simulink library "tqd"  (R2021b)
settings: Solver=VariableStepAuto  StartTime=0.0  StopTime=10.0  RelTol=1e-3
undefined symbols (not defined in the file): ATQD_AfterTqMinGain_X_Deg, ATQD_APSCreepBaseTqD_X_kph, ATQD_APSCreepBaseTqD_Y_Deg, ATQD_APSCreepBaseTqR_X_kph, ATQD_APSCreepBaseTqR_Y_Deg, ATQD_APSCreepIterm_X_kph, ATQD_APSCreepIterm_Y_kph, ATQD_APSCreepPterm_X_kph, ATQD_APSCreepPterm_Y_kph, ATQD_APSDecReq_X_kph, ATQD_APSDecReq_Y_mps2, ATQD_APSDecReqCMD_X_kph, ATQD_APSDecReqTs_X_pct, ATQD_APSDecTimeGain_X_Deg, ATQD_APSDecTimeGain_Y_s, ATQD_APSReqLowSpd_X_Deg, ATQD_AutoHoldReleaseBPS_X_Deg, ATQD_AWDLoadTrqnsGain_X_kg, ATQD_AWDLoadTrqnsGain_Y_pct, ATQD_BOSEnBPSPosn_X_kph, ATQD_BOSMap_X_rpm, ATQD_BOSMap_Y_pct, ATQD_CreepBaseTqD_X_kph, ATQD_CreepBaseTqD_Y_Deg, ATQD_CreepBaseTqR_X_kph, ATQD_CreepBaseTqR_Y_Deg, ATQD_CreepBPSDisPosn_X_Deg, ATQD_CreepBPSDisPosnR_X_Deg, ATQD_CreepBPSEnPosn_X_Deg, ATQD_CreepBPSEnPosnR_X_Deg, ATQD_CreepDeltaTq_X_kph, ATQD_CreepIterm_X_kph, ATQD_CreepIterm_Y_kph, ATQD_CreepItermMaxLimit_X_pct, ATQD_CreepPreloadTime_X_kph, ATQD_CreepPreloadTq_X_kph, ATQD_CreepPreloadTq_Y_s, ATQD_CreepProtTq_X_Deg, ATQD_CreepPterm_X_kph, ATQD_CreepPterm_Y_kph, ATQD_CreepRrTqSpRat_X_rpm, ATQD_CreepRrTqSpRat_Y_Nm, ATQD_CreepTargetSpdD_X_pct, ATQD_CreepTargetSpdR_X_pct, ATQD_ECOTqMapD_X_rpm, ATQD_ECOTqMapD_Y_pct, ATQD_EMTqMapD_X_rpm, ATQD_EMTqMapD_Y_pct, ATQD_EOPDTqMapDCon_X_rpm, ATQD_EOPDTqMapDCon_Y_Deg, ATQD_EscapeModePedTq_X_pct, ATQD_EscapeModePedTq_Y_rpm, ATQD_EscapeModePedTqFr_X_pct, ATQD_EscapeModePedTqFr_Y_rpm, ATQD_EstInitVehWeight_X_c, ATQD_FAfterTqCMDGain_X_rpm, ATQD_FAfterTqCMDGain_Y_pct, ATQD_FrLossMAPLowV_X_rpm, ATQD_FrLossMAPLowV_Y_Nm, ATQD_FrMotActReduce_X_rpm ... (+772)
libraries: simulink x211, hcu_lib x179, tqr x3
(part 27 of 28)

== stateflow chart tqd/TQD/TorqueDemand/Signal_convert/SWC_Subsystem/Speed Control Mode ==
  state OFF
    en:
    VTQD_SpdCtrlMode_enum = ENUM_SPDCTRLMODE_OFF;
    VTQD_SpdCtrlSta_flg = FALSE;
  state ACC
    en:
    VTQD_SpdCtrlMode_enum = ENUM_SPDCTRLMODE_ACC;
    VTQD_SpdCtrlSta_flg = TRUE;
  state CC
    en:
    VTQD_SpdCtrlMode_enum = ENUM_SPDCTRLMODE_CC;
    VTQD_SpdCtrlSta_flg = TRUE;
  state MSA
    en:
    VTQD_SpdCtrlMode_enum = ENUM_SPDCTRLMODE_MSA;
    VTQD_SpdCtrlSta_flg = TRUE;
  state ISA
    en:
    VTQD_SpdCtrlMode_enum = ENUM_SPDCTRLMODE_ISA;
    VTQD_SpdCtrlSta_flg = TRUE;
  (default) -> OFF
  OFF -> (junction 29) [order 2]
  (junction 29) -> (junction 31) : [
      | VPMM_PowerSta_enum == ENUM_POWERSTA_READY &&...
      | VTQD_ShiftGearPosn_enum == ENUM_GEARPOSNTOCAN_D &&...
      | VINP_ADASACCSta_enum != ENUM_ADASACCSTA_OFF &&...
      | VTQD_SpdCtrlShortP_flg]
  (junction 26) -> (junction 93)
  (junction 100) -> (junction 26)
  (junction 40) -> OFF
  (junction 93) -> (junction 40)
  (junction 38) -> (junction 40)
  (junction 36) -> (junction 93)
  OFF -> ACC [order 1] : [
      | VPMM_PowerSta_enum == ENUM_POWERSTA_READY &&...
      | VTQD_ShiftGearPosn_enum == ENUM_GEARPOSNTOCAN_D &&...
      | VINP_ADASACCSta_enum == ENUM_ADASACCSTA_OFF && ...
      | VTQD_SpdCtrlShortP_flg
      | ]
  ACC -> (junction 38) [order 1] : [
      | VPMM_PowerSta_enum != ENUM_POWERSTA_READY ||...
      | VTQD_ShiftGearPosn_enum != ENUM_GEARPOSNTOCAN_D ||...
      | (VINP_ADASACCSta_enum == ENUM_ADASACCSTA_DISABLE ||...
      | VINP_ADASACCSta_enum == ENUM_ADASACCSTA_ERROR) ||...
      | VTQD_SpdCtrlLongP_flg
      | ]
  ACC -> CC [order 2] : [VTQD_SpdCtrlShortP_flg]
  CC -> (junction 36) [order 1] : [
      | VPMM_PowerSta_enum != ENUM_POWERSTA_READY||...
      | VTQD_ShiftGearPosn_enum != ENUM_GEARPOSNTOCAN_D ||...
      | VTQD_SpdCtrlLongP_flg
      | ]
  (junction 31) -> CC
  CC -> (junction 11) [order 2]
  (junction 11) -> (junction 14) [order 2]
  (junction 11) -> MSA [order 1] : [
      | VTQD_SpdCtrlShortP_flg && ...
      | (VINP_ADASISASta_enum == ENUM_ADASISASTA_DISABLE ||...
      | VINP_ADASISASta_enum == ENUM_ADASISASTA_ERROR || ...
      | !VTQD_IVIISAOffsetSpdCHOOSE_flg)
      | %add20230704
      | ]
  (junction 14) -> ISA : [
      | VTQD_SpdCtrlShortP_flg && ...
      | VINP_ADASISASta_enum == ENUM_ADASISASTA_OFF  && ...
      | VTQD_IVIISAOffsetSpdCHOOSE_flg
      | %add20230704
      | ]
  MSA -> ISA [order 2] : [
      | VINP_ADASISASta_enum == ENUM_ADASISASTA_OFF  && ...
      | VTQD_IVIISAOffsetSpdCHOOSE_flg
      | ]
  ISA -> (junction 100) [order 2] : [
      | VINP_ADASISASta_enum == ENUM_ADASISASTA_ERROR || ...
      | VINP_ADASISASta_enum == ENUM_ADASISASTA_DISABLE || ...
      | !VTQD_IVIISAOffsetSpdCHOOSE_flg
      | ]
  (junction 24) -> (junction 100)
  MSA -> (junction 19) [order 1]
  ISA -> (junction 21) [order 1]
  (junction 19) -> (junction 21)
  (junction 21) -> (junction 24) : [VPMM_PowerSta_enum != ENUM_POWERSTA_READY || ...
      | VTQD_ShiftGearPosn_enum != ENUM_GEARPOSNTOCAN_D ||...
      | VTQD_SpdCtrlShortP_flg || ...
      | VTQD_SpdCtrlLongP_flg
      | ]
  data: VPMM_PowerSta_enum input; VTQD_SpdCtrlShortP_flg input; VTQD_SpdCtrlLongP_flg input; ENUM_SPDCTRLMODE_OFF parameter; ENUM_SPDCTRLMODE_ACC parameter; ENUM_SPDCTRLMODE_CC parameter; ENUM_SPDCTRLMODE_ISA parameter; ENUM_SPDCTRLMODE_MSA parameter; FALSE parameter; ENUM_ADASACCSTA_DISABLE parameter; VINP_ADASACCSta_enum input; ENUM_POWERSTA_READY parameter; VINP_ADASISASta_enum input; ENUM_ADASISASTA_DISABLE parameter; VTQD_SpdCtrlMode_enum output uint8; VTQD_SpdCtrlSta_flg output boolean; TRUE parameter; VTQD_IVIISAOffsetSpdCHOOSE_flg input; ENUM_ADASISASTA_ERROR parameter; ENUM_ADASISASTA_OFF parameter; ENUM_ADASACCSTA_ERROR parameter; ENUM_ADASACCSTA_OFF parameter; VTQD_ShiftGearPosn_enum input; ENUM_GEARPOSNTOCAN_D parameter

== stateflow chart tqd/TQD/TorqueDemand/Signal_convert/Regen Level Switch ==
  state OFF
    en:
    VTQD_RegenMode_enum = ENUM_REGENLEVEL_OFF;
  state UserSetting
  state Lv1
    en:
    VTQD_RegenMode_enum = ENUM_REGENLEVEL_LV1;
    VTQD_SaveRegenMode_enum = ENUM_REGENLEVEL_LV1;
  state Lv2
    en:
    VTQD_RegenMode_enum = ENUM_REGENLEVEL_LV2;
    VTQD_SaveRegenMode_enum = ENUM_REGENLEVEL_LV2;
  state Lv3
    en:
    VTQD_RegenMode_enum = ENUM_REGENLEVEL_LV3;
    VTQD_SaveRegenMode_enum = ENUM_REGENLEVEL_LV3;
  state Lv4
    en:
    VTQD_RegenMode_enum = ENUM_REGENLEVEL_LV4;
    VTQD_SaveRegenMode_enum = ENUM_REGENLEVEL_LV4;
  state Lv5
    en:
    VTQD_RegenMode_enum = ENUM_REGENLEVEL_LV5;
    VTQD_SaveRegenMode_enum = ENUM_REGENLEVEL_LV5;
  state One_Pedal_Drive_Mode
    en:
    VTQD_RegenMode_enum = ENUM_REGENLEVEL_OPD;
    VTQD_SaveRegenMode_enum = ENUM_REGENLEVEL_OPD;
  (default) -> OFF : {
      | VTQD_SaveRegenMode_enum = VTQD_ReadRegenMode_enum;
      | }
  Lv1 -> (junction 102) [order 3] : [(VTQD_RegenSWSta_enum == ...
      | ENUM_REGENSWSTA_LONGPRESSUP || ...
      | VINP_SmartEcoModeSW_flg) && ...
      | !VINP_IVISnowModeCmd_flg]
  (junction 102) -> (junction 85)
  (junction 59) -> Lv1 : [VTQD_SaveRegenMode_enum == ENUM_REGENLEVEL_LV1]
  Lv1 -> UserSetting [order 2] : [VTQD_BCMRgnUserEn_flg]
  (junction 56) -> (junction 59) [order 2]
  UserSetting -> Lv1 [order 6] : [VTQD_ActRgnUserSet_enum == ENUM_RGNMODEUSERSET_LV1]
  Lv1 -> OFF [order 1] : [ VPMM_PowerSta_enum != ENUM_POWERSTA_ON && ...
      |  VPMM_PowerSta_enum != ENUM_POWERSTA_READY ]
  Lv1 -> Lv2 [order 4] : [VTQD_RegenSWSta_enum == ...
      | ENUM_REGENSWSTA_SHORTPRESSUP ]
  Lv2 -> Lv1 [order 3] : [VTQD_RegenSWSta_enum == ...
      | ENUM_REGENSWSTA_SHORTPRESSDOWN]
  (junction 56) -> Lv2 [order 1] : [VTQD_SaveRegenMode_enum == ENUM_REGENLEVEL_LV2]
  Lv2 -> (junction 85) [order 4] : [(VTQD_RegenSWSta_enum == ...
      | ENUM_REGENSWSTA_LONGPRESSUP || ...
      | VINP_SmartEcoModeSW_flg) &&...
      | !VINP_IVISnowModeCmd_flg]
  (junction 53) -> (junction 56) [order 2]
  (junction 85) -> (junction 90)
  Lv2 -> UserSetting [order 2] : [VTQD_BCMRgnUserEn_flg]
  Lv2 -> OFF [order 1] : [ VPMM_PowerSta_enum != ENUM_POWERSTA_ON && ...
      |  VPMM_PowerSta_enum != ENUM_POWERSTA_READY ]
  UserSetting -> Lv2 [order 5] : [VTQD_ActRgnUserSet_enum == ENUM_RGNMODEUSERSET_LV2]
  Lv2 -> Lv3 [order 5] : [VTQD_RegenSWSta_enum == ...
      | ENUM_REGENSWSTA_SHORTPRESSUP && ...
      | !VINP_IVISnowModeCmd_flg]
  Lv3 -> Lv2 [order 3] : [VTQD_RegenSWSta_enum == ...
      | ENUM_REGENSWSTA_SHORTPRESSDOWN || ...
      | VINP_IVISnowModeCmd_flg]
  (junction 53) -> Lv3 [order 1] : [VTQD_SaveRegenMode_enum == ENUM_REGENLEVEL_LV3]
  (junction 50) -> (junction 53) [order 2]
  Lv3 -> (junction 90) [order 4] : [(VTQD_RegenSWSta_enum == ...
      | ENUM_REGENSWSTA_LONGPRESSUP || ...
      | VINP_SmartEcoModeSW_flg) && ...
      | !VINP_IVISnowModeCmd_flg]
  (junction 90) -> (junction 95)
  Lv3 -> UserSetting [order 2] : [VTQD_BCMRgnUserEn_flg]
  Lv3 -> OFF [order 1] : [ VPMM_PowerSta_enum != ENUM_POWERSTA_ON && ...
      |  VPMM_PowerSta_enum != ENUM_POWERSTA_READY ]
  UserSetting -> Lv3 [order 4] : [VTQD_ActRgnUserSet_enum == ENUM_RGNMODEUSERSET_LV3]
  Lv3 -> Lv4 [order 5] : [VTQD_RegenSWSta_enum == ...
      | ENUM_REGENSWSTA_SHORTPRESSUP && ...
      | !VINP_IVISnowModeCmd_flg]
  Lv4 -> Lv3 [order 3] : [VTQD_RegenSWSta_enum == ...
      | ENUM_REGENSWSTA_SHORTPRESSDOWN || ...
      | VINP_IVISnowModeCmd_flg]
  (junction 50) -> Lv4 [order 1] : [VTQD_SaveRegenMode_enum == ENUM_REGENLEVEL_LV4]
  Lv4 -> (junction 95) [order 4] : [(VTQD_RegenSWSta_enum == ...
      | ENUM_REGENSWSTA_LONGPRESSUP|| ...
      | VINP_SmartEcoModeSW_flg) && ...
      | !VINP_IVISnowModeCmd_flg ]
  (junction 47) -> (junction 50) [order 2]
  (junction 95) -> (junction 210)
  Lv4 -> UserSetting [order 2] : [VTQD_BCMRgnUserEn_flg]
  UserSetting -> Lv4 [order 3] : [VTQD_ActRgnUserSet_enum == ENUM_RGNMODEUSERSET_LV4]
  Lv4 -> OFF [order 1] : [ VPMM_PowerSta_enum != ENUM_POWERSTA_ON && ...
      |  VPMM_PowerSta_enum != ENUM_POWERSTA_READY ]
  Lv4 -> Lv5 [order 5] : [VTQD_RegenSWSta_enum == ...
      | ENUM_REGENSWSTA_SHORTPRESSUP && ...
      | !VINP_IVISnowModeCmd_flg]
  Lv5 -> Lv4 [order 4] : [VTQD_RegenSWSta_enum == ...
      | ENUM_REGENSWSTA_SHORTPRESSDOWN ||...
      | VINP_IVISnowModeCmd_flg]
  UserSetting -> Lv5 [order 2] : [VTQD_ActRgnUserSet_enum == ENUM_RGNMODEUSERSET_LV5]
  (junction 47) -> Lv5 [order 1] : [VTQD_SaveRegenMode_enum == ENUM_REGENLEVEL_LV5]
  (junction 129) -> (junction 47) [order 2]
  Lv5 -> UserSetting [order 2] : [VTQD_BCMRgnUserEn_flg]
  (junction 210) -> Lv5 [order 1] : [VINP_SmartEcoModeSW_flg && !VINP_IVISnowModeCmd_flg]
  (junction 210) -> (junction 36) [order 2]
  Lv5 -> OFF [order 1] : [ VPMM_PowerSta_enum != ENUM_POWERSTA_ON && ...
      |  VPMM_PowerSta_enum != ENUM_POWERSTA_READY ]
  Lv5 -> (junction 36) [order 3] : [VTQD_RegenSWSta_enum == ...
      | ENUM_REGENSWSTA_LONGPRESSUP && ...
      | !VINP_IVISnowModeCmd_flg && ...
      | !VTQD_TrailerMode_flg && ...
      | !VTQD_OPDModeDis_flg]
      | %add20250215
  (junction 36) -> (junction 39) : [!VTQD_TrailerMode_flg && ...
      |  !VTQD_OPDModeDis_flg]
      | %add20250215
  One_Pedal_Drive_Mode -> Lv5 [order 3] : [VTQD_RegenSWSta_enum == ENUM_REGENSWSTA_SHORTPRESSUP || ...
      |  VTQD_RegenSWSta_enum == ENUM_REGENSWSTA_SHORTPRESSDOWN||...
      |  VINP_IVISnowModeCmd_flg || ...
      |  VTQD_TrailerMode_flg || ...
      |  VTQD_OPDModeDis_flg]
      | %add20250215
  OFF -> (junction 129) [order 2] : [ VPMM_PowerSta_enum == ENUM_POWERSTA_ON || ...
      |  VPMM_PowerSta_enum == ENUM_POWERSTA_READY ]
  (junction 129) -> (junction 205) [order 1]
  OFF -> (junction 220) [order 1] : [VBCM_BCMUserNowSetting_enum != ENUM_BCMUSERNOWSET_INVALID && ...
      |  VBCM_BCMUserNowSetting_enum != ENUM_BCMUSERNOWSET_GUEST && ...
      |  VBCM_BCMUserNowSetting_enum != ENUM_BCMUSERNOWSET_RENT && ...
      |  (VPMM_PowerSta_enum == ENUM_POWERSTA_ON || ...
      |  VPMM_PowerSta_enum == ENUM_POWERSTA_READY)]
      | %add20241217
  (junction 154) -> OFF
  (junction 39) -> One_Pedal_Drive_Mode
  One_Pedal_Drive_Mode -> UserSetting [order 2] : [VTQD_BCMRgnUserEn_flg]
  (junction 205) -> One_Pedal_Drive_Mode : [VTQD_SaveRegenMode_enum == ENUM_REGENLEVEL_OPD]
  One_Pedal_Drive_Mode -> (junction 154) [order 1] : [ VPMM_PowerSta_enum != ENUM_POWERSTA_ON && ...
      |  VPMM_PowerSta_enum != ENUM_POWERSTA_READY ]
  UserSetting -> One_Pedal_Drive_Mode [order 1] : [VTQD_ActRgnUserSet_enum == ENUM_RGNMODEUSERSET_OPD]
  (junction 222) -> UserSetting
  (junction 220) -> (junction 222)
  data: VTQD_RegenMode_enum output uint8 =0; ENUM_REGENLEVEL_LV1 parameter; ENUM_REGENLEVEL_LV2 parameter; ENUM_REGENLEVEL_LV3 parameter; ENUM_REGENLEVEL_LV4 parameter; ENUM_REGENLEVEL_LV5 parameter; ENUM_REGENLEVEL_OPD parameter; VPMM_PowerSta_enum input; ENUM_POWERSTA_ON parameter; ENUM_POWERSTA_READY parameter; VTQD_RegenSWSta_enum input; ENUM_REGENSWSTA_LONGPRESSUP parameter; ENUM_REGENSWSTA_SHORTPRESSDOWN parameter; ENUM_REGENSWSTA_SHORTPRESSUP parameter; ENUM_REGENLEVEL_OFF parameter; VTQD_SaveRegenMode_enum output uint8; VTQD_ReadRegenMode_enum input; VINP_SmartEcoModeSW_flg input; VINP_IVISnowModeCmd_flg input; VTQD_TrailerMode_flg input; VTQD_BCMRgnUserEn_flg input; VTQD_ActRgnUserSet_enum input; VBCM_BCMUserNowSetting_enum input; ENUM_BCMUSERNOWSET_INVALID parameter; ENUM_BCMUSERNOWSET_GUEST parameter; ENUM_BCMUSERNOWSET_RENT parameter; ENUM_RGNMODEUSERSET_LV1 parameter; ENUM_RGNMODEUSERSET_LV2 parameter; ENUM_RGNMODEUSERSET_LV3 parameter; ENUM_RGNMODEUSERSET_LV4 parameter; ENUM_RGNMODEUSERSET_LV5 parameter; ENUM_RGNMODEUSERSET_OPD parameter; VTQD_OPDModeDis_flg input

== stateflow chart tqd/TQD/TorqueDemand/Signal_convert/SWC_Subsystem/Speed Setting Mode/MSA Speed Setting ON/MSA ==
  state MSA
    en:
    VTQD_MSASetSpd_kph = 0;
    VTQD_MSASavedSetSpd_kph = 0;
    state Active
      (default) -> (junction 219)
      (junction 219) -> (junction 220) [order 1] : [VTQD_SWCResUpPress_enum == ENUM_SWCBOTTONPRESS_LONGPRESS  ||...
          |  VTQD_SWCResUpPress_enum == ENUM_SWCBOTTONPRESS_SHORTPRESS ||...
          | VTQD_SWCSetDownPress_enum == ENUM_SWCBOTTONPRESS_LONGPRESS  ||...
          |  VTQD_SWCSetDownPress_enum == ENUM_SWCBOTTONPRESS_SHORTPRESS ]
      (junction 220) -> (junction 221) [order 1] : [VTQD_SWCSetDownPress_enum == ENUM_SWCBOTTONPRESS_LONGPRESS  ||...
          |  VTQD_SWCSetDownPress_enum == ENUM_SWCBOTTONPRESS_SHORTPRESS]
      (junction 219) -> (junction 226) [order 2]
      (junction 220) -> (junction 222) [order 2]
      (junction 221) -> (junction 224)
      (junction 222) -> (junction 223) [order 1] : [VTQD_SWCResUpPress_enum == ENUM_SWCBOTTONPRESS_LONGPRESS]
      (junction 224) -> (junction 225) [order 1] : [VTQD_SWCSetDownPress_enum == ENUM_SWCBOTTONPRESS_LONGPRESS]
      (junction 222) -> (junction 227) [order 2] : %ADD_Short
          | {VTQD_MSASetSpd_kph = VTQD_MSASetSpd_kph + KTQD_SetSpdDeltaShort_kph; ...
          | VTQD_MSASetSpd_kph = min (KTQD_MSAActiveMetSpdHi_raw32,VTQD_MSASetSpd_kph);...
          | VTQD_MSASavedSetSpd_kph = VTQD_MSASetSpd_kph;
          | VTQD_DistanceUnit_flg = VINP_Distanceunit_flg
          | %add20230704
          | }
      (junction 224) -> (junction 229) [order 2] : %SUBSTRACT_Short
          | {VTQD_MSASetSpd_kph = VTQD_MSASetSpd_kph - KTQD_SetSpdDeltaShort_kph; ...
          | VTQD_MSASetSpd_kph = max (KTQD_MSAActiveMetSpdLo_raw32,VTQD_MSASetSpd_kph);...
          | VTQD_MSASavedSetSpd_kph = VTQD_MSASetSpd_kph;
          | VTQD_DistanceUnit_flg = VINP_Distanceunit_flg
          | }
      (junction 223) -> (junction 289)
      (junction 225) -> (junction 296)
      (junction 296) -> (junction 298) [order 1] : [VTQD_SetSpdDeltaLongFit_kph  != 0]
      (junction 296) -> (junction 230) [order 2] : %SUBSTRACT_Long
          | {VTQD_MSASetSpd_kph = VTQD_MSASetSpd_kph - KTQD_SetSpdDeltaLong_kph; ...
          | VTQD_MSASetSpd_kph = max (KTQD_MSAActiveMetSpdLo_raw32,VTQD_MSASetSpd_kph);...
          | VTQD_MSASavedSetSpd_kph = VTQD_MSASetSpd_kph;
          | VTQD_DistanceUnit_flg = VINP_Distanceunit_flg
          | %add20230704
          | }
      (junction 298) -> (junction 300) : {VTQD_MSASetSpd_kph = VTQD_MSASetSpd_kph - VTQD_SetSpdDeltaLongFit_kph; ...
          | VTQD_MSASetSpd_kph = max (KTQD_MSAActiveMetSpdLo_raw32,VTQD_MSASetSpd_kph);...
          | VTQD_MSASavedSetSpd_kph = VTQD_MSASetSpd_kph;
          | VTQD_DistanceUnit_flg = VINP_Distanceunit_flg
          | }
          | %add20231127
      (junction 289) -> (junction 291) [order 1] : [VTQD_SetSpdDeltaLongFit_kph  != 0]
      (junction 289) -> (junction 228) [order 2] : %ADD_Long
          | {VTQD_MSASetSpd_kph = VTQD_MSASetSpd_kph + KTQD_SetSpdDeltaLong_kph; ...
          | VTQD_MSASetSpd_kph = min (KTQD_MSAActiveMetSpdHi_raw32,VTQD_MSASetSpd_kph);...
          | VTQD_MSASavedSetSpd_kph = VTQD_MSASetSpd_kph;
          | VTQD_DistanceUnit_flg = VINP_Distanceunit_flg
          | }
      (junction 291) -> (junction 293) : {VTQD_MSASetSpd_kph = VTQD_MSASetSpd_kph + (KTQD_SetSpdDeltaLongFit_kph-VTQD_SetSpdDeltaLongFit_kph); ...
          | VTQD_MSASetSpd_kph = min (KTQD_MSAActiveMetSpdHi_raw32,VTQD_MSASetSpd_kph);...
          | VTQD_MSASavedSetSpd_kph = VTQD_MSASetSpd_kph;
          | VTQD_DistanceUnit_flg = VINP_Distanceunit_flg
          | %add20231127
          | }
    state OFForDisable
      en:
      VTQD_MSASetSpd_kph = 0;
      VTQD_MSASavedSetSpd_kph = VTQD_MSASetSpd_kph;
      VTQD_DistanceUnit_flg = VINP_Distanceunit_flg
    state ACTIVE_or_STANDBY_CHANGE_TO_OFF
      (default) -> (junction 246)
      (junction 246) -> (junction 247) [order 1] : [VTQD_SWCResUpPress_enum == ENUM_SWCBOTTONPRESS_LONGPRESS  ||...
          |  VTQD_SWCResUpPress_enum == ENUM_SWCBOTTONPRESS_SHORTPRESS ||...
          | VTQD_SWCSetDownPress_enum == ENUM_SWCBOTTONPRESS_LONGPRESS  ||...
          |  VTQD_SWCSetDownPress_enum == ENUM_SWCBOTTONPRESS_SHORTPRESS   ]
      (junction 247) -> (junction 248) [order 1] : [VTQD_SWCResUpPress_enum == ENUM_SWCBOTTONPRESS_LONGPRESS  ||...
          |  VTQD_SWCResUpPress_enum == ENUM_SWCBOTTONPRESS_SHORTPRESS]
      (junction 247) -> (junction 250) [order 2] : {VTQD_MSASetSpd_kph = VVMC_MeterIndSpeed_raw32;
          | VTQD_MSASavedSetSpd_kph=VVMC_MeterIndSpeed_raw32;
          | VTQD_MSASetSpd_kph = max (KTQD_MSAActiveMetSpdLo_raw32,VTQD_MSASetSpd_kph);
          | VTQD_MSASavedSetSpd_kph = VTQD_MSASetSpd_kph;;
          | VTQD_DistanceUnit_flg = VINP_Distanceunit_flg
          | }
          | %add20231127
      (junction 248) -> (junction 251) : {VTQD_MSASetSpd_kph = VTQD_MSASavedSetSpd_kph
          | VTQD_MSASavedSetSpd_kph = VTQD_MSASetSpd_kph;;
          | VTQD_DistanceUnit_flg = VINP_Distanceunit_flg}
      (junction 246) -> (junction 249) [order 2]
    state LoopBack
    state SetDown
    (default) -> (junction 188) : {VTQD_DistanceUnit_flg = VINP_Distanceunit_flg}
    (junction 320) -> (junction 307) [order 1] : [VTQD_DistanceUnit_flg == VINP_Distanceunit_flg || VTQD_MSASavedSetSpd_kph <= ONE_FLOAT]
    MSA -> (junction 320)
    (junction 307) -> (junction 188) : {VTQD_MSASetSpd_kph = min (KTQD_MSAActiveMetSpdHi_raw32,VTQD_MSASetSpd_kph);
        | VTQD_MSASavedSetSpd_kph = VTQD_MSASetSpd_kph;}
    (junction 320) -> (junction 306) [order 2]
    (junction 314) -> (junction 307)
    (junction 188) -> (junction 190)
    (junction 306) -> (junction 310) [order 1] : [VINP_Distanceunit_flg == TRUE]
    (junction 306) -> (junction 364) [order 2] : {VTQD_MSASavedSetSpd_kph = (VTQD_MSASavedSetSpd_kph * MPH2KPH)}
    (junction 310) -> (junction 365) : {VTQD_MSASavedSetSpd_kph = (VTQD_MSASavedSetSpd_kph * KPH2MPH)}
    (junction 190) -> (junction 191) [order 1] : [VVMC_MSACrlSta_enum == ENUM_ADASMSASTA_UNDERSPEED ||...
        |  VVMC_MSACrlSta_enum == ENUM_ADASMSASTA_OVERSPEED ||...
        | VVMC_MSACrlSta_enum == ENUM_ADASMSASTA_ERROR ||...
        |  VVMC_MSACrlSta_enum == ENUM_ADASMSASTA_INVAILD  ||...
        |  VVMC_MSACrlSta_enum == ENUM_ADASMSASTA_OFF] %W Add
    (junction 190) -> (junction 192) [order 2]
    (junction 191) -> OFForDisable
    (junction 192) -> (junction 193) [order 1] : [VVMC_MSACrlSta_enum == ENUM_ADASMSASTA_ACTIVE]
        | %W Delete || VINP_MSACrlSta_enum == ENUM_ADASMSASTA_STANDBY]
    (junction 192) -> (junction 194) [order 2]
    (junction 193) -> Active : {VTQD_MSASetSpd_kph = VTQD_MSASavedSetSpd_kph;
        | VTQD_MSASavedSetSpd_kph = VTQD_MSASetSpd_kph;;
        | VTQD_DistanceUnit_flg = VINP_Distanceunit_flg}
    (junction 364) -> (junction 346) [order 1] : [VTQD_MSASavedSetSpd_kph < KTQD_MSAActiveMetSpdLo_kph]
    (junction 365) -> (junction 332) [order 1] : [VTQD_MSASavedSetSpd_kph < KTQD_MSAActiveMetSpdLoMPH_mph]
    (junction 364) -> (junction 348) [order 2]
    (junction 346) -> (junction 345) : {VTQD_MSASavedSetSpd_kph = KTQD_MSAActiveMetSpdLo_kph}
    (junction 365) -> (junction 336) [order 2]
    (junction 332) -> (junction 333) : {VTQD_MSASavedSetSpd_kph = KTQD_MSAActiveMetSpdLoMPH_mph}
    (junction 194) -> (junction 195) [order 1] : [VVMC_MSACrlSta_enum == ENUM_ADASMSASTA_UNLIMIT ||...
        |  VVMC_MSACrlSta_enum == ENUM_ADASMSASTA_STANDBY] %W Add
        |  %W Delete  ||  VINP_MSACrlSta_enum == ENUM_ADASMSASTA_OFF
        | %add 20231127
    (junction 195) -> (junction 196) [order 1] : [VTQD_ChangeToOFF_flg]
    (junction 333) -> (junction 336)
    (junction 345) -> (junction 348)
    (junction 194) -> LoopBack [order 2] : {VTQD_MSASetSpd_kph = VTQD_MSASavedSetSpd_kph;
        | VTQD_MSASavedSetSpd_kph = VTQD_MSASetSpd_kph;;
        | VTQD_DistanceUnit_flg = VINP_Distanceunit_flg}
    (junction 195) -> (junction 197) [order 2]
    (junction 196) -> ACTIVE_or_STANDBY_CHANGE_TO_OFF : {VTQD_MSASetSpd_kph = VTQD_MSASavedSetSpd_kph;
        | VTQD_MSASavedSetSpd_kph = VTQD_MSASetSpd_kph;;
        | VTQD_DistanceUnit_flg = VINP_Distanceunit_flg}
    (junction 336) -> (junction 344)
    (junction 348) -> (junction 354)
    (junction 354) -> (junction 352) [order 1] : [VTQD_MSASavedSetSpd_kph > KTQD_MSAActiveMetSpdHi_kph]
    (junction 344) -> (junction 340) [order 1] : [VTQD_MSASavedSetSpd_kph > KTQD_MSAActiveMetSpdHiMPH_mph]
    (junction 354) -> (junction 357) [order 2]
    (junction 352) -> (junction 353) : {VTQD_MSASavedSetSpd_kph = KTQD_MSAActiveMetSpdHi_kph}
    (junction 344) -> (junction 341) [order 2]
    (junction 340) -> (junction 343) : {VTQD_MSASavedSetSpd_kph = KTQD_MSAActiveMetSpdHiMPH_mph}
    (junction 197) -> (junction 198) [order 1] : [VTQD_SWCSetDownPress_enum == ENUM_SWCBOTTONPRESS_LONGPRESS  ||...
        |  VTQD_SWCSetDownPress_enum == ENUM_SWCBOTTONPRESS_SHORTPRESS  ]
    (junction 197) -> LoopBack [order 2] : {VTQD_MSASetSpd_kph = VTQD_MSASavedSetSpd_kph;
        | VTQD_MSASavedSetSpd_kph = VTQD_MSASetSpd_kph;;
        | VTQD_DistanceUnit_flg = VINP_Distanceunit_flg}
    (junction 198) -> SetDown : {VTQD_MSASetSpd_kph = VVMC_MeterIndSpeed_raw32;
        | VTQD_MSASavedSetSpd_kph=VVMC_MeterIndSpeed_raw32;
        | VTQD_MSASetSpd_kph = max (KTQD_MSAActiveMetSpdLo_raw32,VTQD_MSASetSpd_kph);
        | VTQD_MSASavedSetSpd_kph = VTQD_MSASetSpd_kph;;
        | VTQD_DistanceUnit_flg = VINP_Distanceunit_flg}
        | %add20231118
    (junction 353) -> (junction 357)
    (junction 343) -> (junction 341)
    (junction 357) -> (junction 312)
    (junction 341) -> (junction 311)
    (junction 312) -> (junction 311)
    (junction 311) -> (junction 314)
  data: KTQD_SetSpdDeltaLong_kph input; KTQD_SetSpdDeltaShort_kph input; VTQD_SWCSetDownPress_enum input; VINP_Distanceunit_flg input; VTQD_ChangeToOFF_flg input; VVMC_MeterIndSpeed_raw32 input; KTQD_MSAActiveMetSpdHi_raw32 input; KTQD_MSAActiveMetSpdLo_raw32 input; VVMC_MSACrlSta_enum input; VTQD_SetSpdDeltaLongFit_kph input; KTQD_SetSpdDeltaLongFit_kph input; VTQD_MSASavedSetSpd_kph local double; ENUM_ADASMSASTA_ACTIVE parameter; ENUM_ADASMSASTA_ERROR parameter; ENUM_ADASMSASTA_INVAILD parameter; ENUM_ADASMSASTA_OFF parameter; ENUM_ADASMSASTA_OVERSPEED parameter; ENUM_ADASMSASTA_STANDBY parameter; ENUM_ADASMSASTA_UNDERSPEED parameter; VTQD_MSASetSpd_kph output single; ENUM_SWCBOTTONPRESS_LONGPRESS parameter; ENUM_SWCBOTTONPRESS_SHORTPRESS parameter; VTQD_SWCResUpPress_enum input; ENUM_ADASMSASTA_UNLIMIT parameter; KPH2MPH parameter; MPH2KPH parameter; TRUE parameter; VTQD_DistanceUnit_flg local boolean; ONE_FLOAT parameter; KTQD_MSAActiveMetSpdHiMPH_mph parameter; KTQD_MSAActiveMetSpdLoMPH_mph parameter; KTQD_MSAActiveMetSpdLo_kph parameter; KTQD_MSAActiveMetSpdHi_kph parameter

== stateflow chart tqd/TQD/TorqueDemand/Signal_convert/SWC_Subsystem/Speed Setting Mode/MSA Speed Setting ON/Specific_STATE_ChangeToOFF ==
  state FLG_ON
    en:
    VTQD_ChangeToOFF_flg = TRUE;
  state Initialize
    en:
    VTQD_ChangeToOFF_flg = FALSE;
  state STAY
  (default) -> Initialize
  Initialize -> STAY : [VINP_MSACrlSta_enum == ENUM_ADASMSASTA_UNLIMIT ||...
      | VINP_MSACrlSta_enum == ENUM_ADASMSASTA_ACTIVE]
  STAY -> FLG_ON [order 1] : [VINP_MSACrlSta_enum == ENUM_ADASMSASTA_STANDBY]
  STAY -> Initialize [order 2] : [VINP_MSACrlSta_enum != ENUM_ADASMSASTA_STANDBY &&...
      | VINP_MSACrlSta_enum != ENUM_ADASMSASTA_ACTIVE&&...
      | VINP_MSACrlSta_enum != ENUM_ADASMSASTA_UNLIMIT]
  (junction 11) -> Initialize
  FLG_ON -> (junction 9)
  (junction 9) -> (junction 11) : [VINP_MSACrlSta_enum != ENUM_ADASMSASTA_STANDBY]
  data: VINP_MSACrlSta_enum input; VTQD_ChangeToOFF_flg output boolean; FALSE parameter; TRUE parameter; ENUM_ADASMSASTA_ACTIVE parameter; ENUM_ADASMSASTA_STANDBY parameter; ENUM_ADASMSASTA_UNLIMIT parameter

== stateflow chart tqd/TQD/TorqueDemand/Signal_convert/SWC2_Subsystem/Speed Setting Mode/CC Speed Setting ON/CC Speed Setting Mode ==
  state CC
    en:
    VTQD_CCSetSpd_kph = 0;
    VTQD_CCSavedSetSpd_kph = 0;
    VTQD_CCSpdResetFinish_flg = 0;
    state Active
      (default) -> (junction 61)
      (junction 61) -> (junction 65) [order 1] : [VTQD_SWCResUpPress_enum == ENUM_SWCBOTTONPRESS_LONGPRESS  ||...
          |  VTQD_SWCResUpPress_enum == ENUM_SWCBOTTONPRESS_SHORTPRESS ||...
          | VTQD_SWCSetDownPress_enum == ENUM_SWCBOTTONPRESS_LONGPRESS  ||...
          |  VTQD_SWCSetDownPress_enum == ENUM_SWCBOTTONPRESS_SHORTPRESS   ]
      (junction 65) -> (junction 69) [order 1] : [VTQD_SWCSetDownPress_enum == ENUM_SWCBOTTONPRESS_LONGPRESS  ||...
          |  VTQD_SWCSetDownPress_enum == ENUM_SWCBOTTONPRESS_SHORTPRESS ]
      (junction 61) -> (junction 63) [order 2]
      (junction 65) -> (junction 67) [order 2]
      (junction 69) -> (junction 80)
      (junction 67) -> (junction 71) [order 1] : [VTQD_SWCResUpPress_enum == ENUM_SWCBOTTONPRESS_LONGPRESS]
      (junction 80) -> (junction 82) [order 1] : [VTQD_SWCSetDownPress_enum == ENUM_SWCBOTTONPRESS_LONGPRESS]
      (junction 67) -> (junction 73) [order 2] : %ADD_Short
          | {VTQD_CCSetSpd_kph = VTQD_CCSetSpd_kph + KTQD_SetSpdDeltaShort_kph; ...
          | VTQD_CCSetSpd_kph = min (KTQD_CCActiveMetSpdHi_raw32,VTQD_CCSetSpd_kph);...
          | VTQD_CCSavedSetSpd_kph = VTQD_CCSetSpd_kph;
          | VTQD_DistanceUnit_flg = VINP_Distanceunit_flg
          | }
      (junction 80) -> (junction 83) [order 2] : %SUBSTRACT_Short
          | {VTQD_CCSetSpd_kph = VTQD_CCSetSpd_kph - KTQD_SetSpdDeltaShort_kph; ...
          | VTQD_CCSetSpd_kph = max (KTQD_CCActiveMetSpdLo_raw32,VTQD_CCSetSpd_kph);...
          | VTQD_CCSavedSetSpd_kph = VTQD_CCSetSpd_kph;
          | VTQD_DistanceUnit_flg = VINP_Distanceunit_flg
          | }
      (junction 71) -> (junction 272)
      (junction 82) -> (junction 278)
      (junction 272) -> (junction 274) [order 1] : [VTQD_SetSpdDeltaLongFit_kph != 0]
      (junction 278) -> (junction 282) [order 1] : [VTQD_SetSpdDeltaLongFit_kph != 0]
      (junction 272) -> (junction 75) [order 2] : %ADD_Long
          | {VTQD_CCSetSpd_kph = VTQD_CCSetSpd_kph + KTQD_SetSpdDeltaLong_kph; ...
          | VTQD_CCSetSpd_kph = min (KTQD_CCActiveMetSpdHi_raw32,VTQD_CCSetSpd_kph);...
          | VTQD_CCSavedSetSpd_kph = VTQD_CCSetSpd_kph;
          | VTQD_DistanceUnit_flg = VINP_Distanceunit_flg
          | }
      (junction 274) -> (junction 276) : {
          | VTQD_CCSetSpd_kph = VTQD_CCSetSpd_kph + (KTQD_SetSpdDeltaLongFit_kph-VTQD_SetSpdDeltaLongFit_kph); ...
          | VTQD_CCSetSpd_kph = min (KTQD_CCActiveMetSpdHi_raw32,VTQD_CCSetSpd_kph); ...
          | VTQD_CCSavedSetSpd_kph = VTQD_CCSetSpd_kph;
          | VTQD_DistanceUnit_flg = VINP_Distanceunit_flg
          | }
          | %add20231127
      (junction 278) -> (junction 85) [order 2] : %SUBSTRACT_Long
          | {VTQD_CCSetSpd_kph = VTQD_CCSetSpd_kph - KTQD_SetSpdDeltaLong_kph; ...
          | VTQD_CCSetSpd_kph = max (KTQD_CCActiveMetSpdLo_raw32,VTQD_CCSetSpd_kph);...
          | VTQD_CCSavedSetSpd_kph = VTQD_CCSetSpd_kph;
          | VTQD_DistanceUnit_flg = VINP_Distanceunit_flg
          | }
      (junction 282) -> (junction 284) : {VTQD_CCSetSpd_kph = VTQD_CCSetSpd_kph - VTQD_SetSpdDeltaLongFit_kph; ...
          | VTQD_CCSetSpd_kph = max (KTQD_CCActiveMetSpdLo_raw32,VTQD_CCSetSpd_kph);...
          | VTQD_CCSavedSetSpd_kph = VTQD_CCSetSpd_kph;
          | VTQD_DistanceUnit_flg = VINP_Distanceunit_flg}
          | %add20231122
    state OFForDisable
      en:
      VTQD_CCSetSpd_kph = 0;
      VTQD_CCSavedSetSpd_kph=VTQD_CCSetSpd_kph;
      VTQD_DistanceUnit_flg = VINP_Distanceunit_flg
    state ChangeFrom_ACTIVE
      (default) -> (junction 238)
      (junction 238) -> (junction 239) [order 1] : [VTQD_CCSpdResetFinish_flg]
      (junction 238) -> (junction 241) [order 2] : {VTQD_CCSetSpd_kph = VTQD_CCSavedSetSpd_kph;}
          | %add20231206
      (junction 239) -> (junction 244)
      (junction 244) -> (junction 241)
      (junction 241) -> (junction 206)
      (junction 206) -> (junction 203) [order 1] : [VTQD_SWCResUpPress_enum == ENUM_SWCBOTTONPRESS_LONGPRESS  ||...
          |  VTQD_SWCResUpPress_enum == ENUM_SWCBOTTONPRESS_SHORTPRESS ||...
          | VTQD_SWCSetDownPress_enum == ENUM_SWCBOTTONPRESS_LONGPRESS  ||...
          |  VTQD_SWCSetDownPress_enum == ENUM_SWCBOTTONPRESS_SHORTPRESS   ]
      (junction 203) -> (junction 205) [order 1] : [VTQD_SWCResUpPress_enum == ENUM_SWCBOTTONPRESS_LONGPRESS  ||...
          |  VTQD_SWCResUpPress_enum == ENUM_SWCBOTTONPRESS_SHORTPRESS ]
      (junction 203) -> (junction 209) [order 2] : {VTQD_CCSetSpd_kph = VVMC_MeterIndSpeed_raw32;
          | VTQD_CCSpdResetFinish_flg = TRUE;
          | VTQD_CCSetSpd_kph = max (KTQD_CCActiveMetSpdLo_raw32,VTQD_CCSetSpd_kph);
          | VTQD_CCSavedSetSpd_kph=VTQD_CCSetSpd_kph;
          | VTQD_DistanceUnit_flg = VINP_Distanceunit_flg}
          | %add20231206
      (junction 206) -> (junction 211) [order 2]
      (junction 205) -> (junction 210) : {VTQD_CCSetSpd_kph = VTQD_CCSavedSetSpd_kph;
          | VTQD_CCSpdResetFinish_flg = TRUE;
          | VTQD_CCSavedSetSpd_kph=VTQD_CCSetSpd_kph;
          | VTQD_DistanceUnit_flg = VINP_Distanceunit_flg}
    state SetDown
    state LoopBack
    (default) -> (junction 1) : {VTQD_DistanceUnit_flg = VINP_Distanceunit_flg}
    (junction 1) -> (junction 3) [order 1] : [VVMC_CCCtrlSta_enum != ENUM_ADASCCSTA_STANDBY &&...
        |  VVMC_CCCtrlSta_enum != ENUM_ADASCCSTA_ACTIVE &&...
        |  VVMC_CCCtrlSta_enum != ENUM_ADASCCSTA_OVRRIDE]
    CC -> (junction 253)
    (junction 253) -> (junction 258) [order 2]
    (junction 258) -> (junction 300)
    (junction 300) -> (junction 290) [order 1] : [VTQD_DistanceUnit_flg == VINP_Distanceunit_flg || VTQD_CCSavedSetSpd_kph <= ONE_FLOAT]
    (junction 290) -> (junction 1) : {VTQD_CCSetSpd_kph = min (KTQD_CCActiveMetSpdHi_raw32,VTQD_CCSetSpd_kph);
        | VTQD_CCSavedSetSpd_kph = VTQD_CCSetSpd_kph;}
        | %add20240918
    (junction 300) -> (junction 289) [order 2]
    (junction 1) -> (junction 20) [order 2]
    (junction 3) -> OFForDisable
    (junction 253) -> (junction 255) [order 1]
    (junction 256) -> (junction 258) : {VTQD_CCSpdResetFinish_flg = FALSE;}
    (junction 292) -> (junction 290)
    (junction 289) -> (junction 295) [order 1] : [VINP_Distanceunit_flg == TRUE]
    (junction 289) -> (junction 340) [order 2] : {VTQD_CCSavedSetSpd_kph = (VTQD_CCSavedSetSpd_kph * MPH2KPH)}
    (junction 295) -> (junction 342) : {VTQD_CCSavedSetSpd_kph = (VTQD_CCSavedSetSpd_kph * KPH2MPH)}
    (junction 255) -> (junction 256) : [VVMC_CCCtrlSta_enum != ENUM_ADASCCSTA_STANDBY &&...
        | VTQD_CCSpdResetFinish_flg]
    (junction 20) -> (junction 228) [order 1] : [VVMC_CCCtrlSta_enum == ENUM_ADASCCSTA_ACTIVE ||...
        | VVMC_CCCtrlSta_enum == ENUM_ADASCCSTA_OVRRIDE
        | ]
    (junction 228) -> (junction 25) [order 2]
    (junction 20) -> (junction 181) [order 2]
    (junction 228) -> (junction 28) [order 1] : [VVMC_CCCtrlSta_enum == ENUM_ADASCCSTA_OVRRIDE]
    (junction 25) -> Active : {VTQD_CCSetSpd_kph = VTQD_CCSavedSetSpd_kph;
        | VTQD_CCSavedSetSpd_kph=VTQD_CCSetSpd_kph;
        | VTQD_DistanceUnit_flg = VINP_Distanceunit_flg}
    (junction 340) -> (junction 323) [order 1] : [VTQD_CCSavedSetSpd_kph < KTQD_CCActiveMetSpdLo_kph]
    (junction 342) -> (junction 311) [order 1] : [VTQD_CCSavedSetSpd_kph < KTQD_CCActiveMetSpdLoMPH_mph]
    (junction 340) -> (junction 324) [order 2]
    (junction 323) -> (junction 326) : {VTQD_CCSavedSetSpd_kph = KTQD_CCActiveMetSpdLo_kph}
    (junction 342) -> (junction 321) [order 2]
    (junction 311) -> (junction 307) : {VTQD_CCSavedSetSpd_kph = KTQD_CCActiveMetSpdLoMPH_mph}
    (junction 181) -> (junction 28) [order 1] : [VVMC_CCCtrlSta_enum == ENUM_ADASCCSTA_STANDBY]
    (junction 28) -> (junction 40) [order 1] : [VTQD_ChangeToSTANDBY_flg]
    (junction 181) -> LoopBack [order 2] : {VTQD_CCSetSpd_kph = VTQD_CCSavedSetSpd_kph;
        | VTQD_CCSavedSetSpd_kph=VTQD_CCSetSpd_kph;
        | VTQD_DistanceUnit_flg = VINP_Distanceunit_flg}
    (junction 28) -> (junction 43) [order 2]
    (junction 40) -> ChangeFrom_ACTIVE : {VTQD_CCSetSpd_kph = VTQD_CCSavedSetSpd_kph;
        | VTQD_CCSavedSetSpd_kph=VTQD_CCSetSpd_kph;
        | VTQD_DistanceUnit_flg = VINP_Distanceunit_flg}
    (junction 307) -> (junction 321)
    (junction 326) -> (junction 324)
    (junction 321) -> (junction 318)
    (junction 324) -> (junction 330)
    (junction 330) -> (junction 328) [order 1] : [VTQD_CCSavedSetSpd_kph > KTQD_CCActiveMetSpdHi_kph]
    (junction 318) -> (junction 313) [order 1] : [VTQD_CCSavedSetSpd_kph > KTQD_CCActiveMetSpdHiMPH_mph]
    (junction 330) -> (junction 334) [order 2]
    (junction 328) -> (junction 331) : {VTQD_CCSavedSetSpd_kph = KTQD_CCActiveMetSpdHi_kph}
    (junction 318) -> (junction 320) [order 2]
    (junction 313) -> (junction 316) : {VTQD_CCSavedSetSpd_kph = KTQD_CCActiveMetSpdHiMPH_mph}
    (junction 43) -> (junction 44) [order 1] : [VTQD_SWCSetDownPress_enum == ENUM_SWCBOTTONPRESS_LONGPRESS  ||...
        |  VTQD_SWCSetDownPress_enum == ENUM_SWCBOTTONPRESS_SHORTPRESS ]
    (junction 43) -> LoopBack [order 2] : {VTQD_CCSetSpd_kph = VTQD_CCSavedSetSpd_kph;
        | VTQD_CCSavedSetSpd_kph=VTQD_CCSetSpd_kph;
        | VTQD_DistanceUnit_flg = VINP_Distanceunit_flg}
    (junction 44) -> SetDown : {VTQD_CCSetSpd_kph = VVMC_MeterIndSpeed_raw32;
        | VTQD_CCSetSpd_kph = max (KTQD_CCActiveMetSpdLo_raw32,VTQD_CCSetSpd_kph);
        | VTQD_CCSavedSetSpd_kph=VTQD_CCSetSpd_kph;
        | VTQD_DistanceUnit_flg = VINP_Distanceunit_flg}
        | %add20231201
    (junction 331) -> (junction 334)
    (junction 316) -> (junction 320)
    (junction 334) -> (junction 301)
    (junction 320) -> (junction 291)
    (junction 301) -> (junction 291)
    (junction 291) -> (junction 292)
  data: KTQD_SetSpdDeltaLong_kph input; KTQD_SetSpdDeltaShort_kph input; KTQD_SetSpdDeltaLongFit_kph input; VTQD_SetSpdDeltaLongFit_kph input; VVMC_CCCtrlSta_enum input; VINP_Distanceunit_flg input; KTQD_CCActiveMetSpdHi_raw32 input; KTQD_CCActiveMetSpdLo_raw32 input; VVMC_MeterIndSpeed_raw32 input; VTQD_CCSetSpd_kph output single; VTQD_CCSavedSetSpd_kph local single; ENUM_ADASCCSTA_ACTIVE parameter; ENUM_ADASCCSTA_STANDBY parameter; VTQD_SWCSetDownPress_enum input; VTQD_SWCResUpPress_enum input; VTQD_ChangeToSTANDBY_flg input; ENUM_ADASCCSTA_OVRRIDE parameter; VTQD_CCSpdResetFinish_flg output; ENUM_SWCBOTTONPRESS_LONGPRESS parameter; ENUM_SWCBOTTONPRESS_SHORTPRESS parameter; FALSE parameter; TRUE parameter; KPH2MPH parameter; MPH2KPH parameter; VTQD_DistanceUnit_flg local boolean; ONE_FLOAT parameter; KTQD_CCActiveMetSpdHiMPH_mph parameter; KTQD_CCActiveMetSpdHi_kph parameter; KTQD_CCActiveMetSpdLoMPH_mph parameter; KTQD_CCActiveMetSpdLo_kph parameter

== stateflow chart tqd/TQD/TorqueDemand/Signal_convert/SWC2_Subsystem/Speed Setting Mode/CC Speed Setting ON/Specific_STATE_ChangeToSTANDBY ==
  state FLG_ON
    en:
    VTQD_CCChangeToSTANDBY_flg = TRUE;
  state Initialize
    en:
    VTQD_CCChangeToSTANDBY_flg = FALSE;
  state STAY
  (default) -> Initialize
  Initialize -> STAY : [VVMC_CCCtrlSta_enum == ENUM_ADASCCSTA_ACTIVE]
  STAY -> FLG_ON [order 1] : [VVMC_CCCtrlSta_enum == ENUM_ADASCCSTA_STANDBY]
  STAY -> Initialize [order 2] : [VVMC_CCCtrlSta_enum != ENUM_ADASCCSTA_ACTIVE &&...
      | VVMC_CCCtrlSta_enum != ENUM_ADASCCSTA_STANDBY ]
  (junction 11) -> Initialize
  FLG_ON -> (junction 9)
  (junction 9) -> (junction 11) : [VVMC_CCCtrlSta_enum != ENUM_ADASCCSTA_STANDBY]
  data: VVMC_CCCtrlSta_enum input; FALSE parameter; TRUE parameter; VTQD_CCChangeToSTANDBY_flg output boolean; ENUM_ADASCCSTA_ACTIVE parameter; ENUM_ADASCCSTA_STANDBY parameter
